simulink model "ass"  (Simulink 6.5)
settings: Solver=ode45  StartTime=0.0  StopTime=10.0  RelTol=1e-3
libraries: cdsFilt x333, cdsPhase x144, cdsRfmIO x26, cdsOsc x18, cdsMuxMatrix x8, cdsEpicsOut x3, cdsEzCaRead x1, cdsEpicsIn x1, cdsBitwise x1, cdsParameters x1
(part 12 of 17)

== system ass/PIT1/PD2_X/F3 ==
  In1 : Inport
  In2 : Inport  Port=2
  In3 : Inport  Port=3
  I : cdsFilt/Subsystem  Tag=cdsFilt  Description=|  SystemSampleTime=-1
      | Purpose:                                                                                                                                                                                                                                  
      | Standard CDS IIR filter module.                                                                                                                                                                                                           
      |                                                                                                                                                                                                                                           
      | Operation:                                                                                                                                                                                                                                
      | Consists of 10 second order section IIR filters, plus a ramped gain stage. In FE code, also provides pre-defined test points and excitation channel inputs. The filter coefficients are defined in the LIGO system using the 'foton' tool.
      |                                                                                                                                                                                                                                           
      | Usage:                                                                                                                                                                                                                                    
      | Name the part with the desired filter module name.
      settings: AttributesFormatString=%<Tag>
  PHASE : cdsPhase/Subsystem  Tag=cdsPhase  Description=Phase Rotator  SystemSampleTime=-1
      settings: AttributesFormatString=%<Tag>
  Product : Product  RndMeth=Zero
  Product1 : Product  RndMeth=Zero
  Q : cdsFilt/Subsystem  Tag=cdsFilt  Description=|  SystemSampleTime=-1
      | Purpose:                                                                                                                                                                                                                                  
      | Standard CDS IIR filter module.                                                                                                                                                                                                           
      |                                                                                                                                                                                                                                           
      | Operation:                                                                                                                                                                                                                                
      | Consists of 10 second order section IIR filters, plus a ramped gain stage. In FE code, also provides pre-defined test points and excitation channel inputs. The filter coefficients are defined in the LIGO system using the 'foton' tool.
      |                                                                                                                                                                                                                                           
      | Usage:                                                                                                                                                                                                                                    
      | Name the part with the desired filter module name.
      settings: AttributesFormatString=%<Tag>
  Terminator4 : Terminator
  Out1 : Outport
  wires:
  I/1 -> Out1/1
  PHASE/2 -> Q/1
  In1/1 -> Product/1, Product1/1
  In2/1 -> Product/2
  In3/1 -> Product1/2
  PHASE/1 -> I/1
  Product/1 -> PHASE/1
  Q/1 -> Terminator4/1
  Product1/1 -> PHASE/2

== system ass/PIT1/PD2_X/F4 ==
  In1 : Inport
  In2 : Inport  Port=2
  In3 : Inport  Port=3
  I : cdsFilt/Subsystem  Tag=cdsFilt  Description=|  SystemSampleTime=-1
      | Purpose:                                                                                                                                                                                                                                  
      | Standard CDS IIR filter module.                                                                                                                                                                                                           
      |                                                                                                                                                                                                                                           
      | Operation:                                                                                                                                                                                                                                
      | Consists of 10 second order section IIR filters, plus a ramped gain stage. In FE code, also provides pre-defined test points and excitation channel inputs. The filter coefficients are defined in the LIGO system using the 'foton' tool.
      |                                                                                                                                                                                                                                           
      | Usage:                                                                                                                                                                                                                                    
      | Name the part with the desired filter module name.
      settings: AttributesFormatString=%<Tag>
  PHASE : cdsPhase/Subsystem  Tag=cdsPhase  Description=Phase Rotator  SystemSampleTime=-1
      settings: AttributesFormatString=%<Tag>
  Product : Product  RndMeth=Zero
  Product1 : Product  RndMeth=Zero
  Q : cdsFilt/Subsystem  Tag=cdsFilt  Description=|  SystemSampleTime=-1
      | Purpose:                                                                                                                                                                                                                                  
      | Standard CDS IIR filter module.                                                                                                                                                                                                           
      |                                                                                                                                                                                                                                           
      | Operation:                                                                                                                                                                                                                                
      | Consists of 10 second order section IIR filters, plus a ramped gain stage. In FE code, also provides pre-defined test points and excitation channel inputs. The filter coefficients are defined in the LIGO system using the 'foton' tool.
      |                                                                                                                                                                                                                                           
      | Usage:                                                                                                                                                                                                                                    
      | Name the part with the desired filter module name.
      settings: AttributesFormatString=%<Tag>
  Terminator4 : Terminator
  Out1 : Outport
  wires:
  I/1 -> Out1/1
  PHASE/2 -> Q/1
  In1/1 -> Product/1, Product1/1
  In2/1 -> Product/2
  In3/1 -> Product1/2
  PHASE/1 -> I/1
  Product/1 -> PHASE/1
  Q/1 -> Terminator4/1
  Product1/1 -> PHASE/2

== system ass/PIT1/PD2_X/F5 ==
  In1 : Inport
  In2 : Inport  Port=2
  In3 : Inport  Port=3
  I : cdsFilt/Subsystem  Tag=cdsFilt  Description=|  SystemSampleTime=-1
      | Purpose:                                                                                                                                                                                                                                  
      | Standard CDS IIR filter module.                                                                                                                                                                                                           
      |                                                                                                                                                                                                                                           
      | Operation:                                                                                                                                                                                                                                
      | Consists of 10 second order section IIR filters, plus a ramped gain stage. In FE code, also provides pre-defined test points and excitation channel inputs. The filter coefficients are defined in the LIGO system using the 'foton' tool.
      |                                                                                                                                                                                                                                           
      | Usage:                                                                                                                                                                                                                                    
      | Name the part with the desired filter module name.
      settings: AttributesFormatString=%<Tag>
  PHASE : cdsPhase/Subsystem  Tag=cdsPhase  Description=Phase Rotator  SystemSampleTime=-1
      settings: AttributesFormatString=%<Tag>
  Product : Product  RndMeth=Zero
  Product1 : Product  RndMeth=Zero
  Q : cdsFilt/Subsystem  Tag=cdsFilt  Description=|  SystemSampleTime=-1
      | Purpose:                                                                                                                                                                                                                                  
      | Standard CDS IIR filter module.                                                                                                                                                                                                           
      |                                                                                                                                                                                                                                           
      | Operation:                                                                                                                                                                                                                                
      | Consists of 10 second order section IIR filters, plus a ramped gain stage. In FE code, also provides pre-defined test points and excitation channel inputs. The filter coefficients are defined in the LIGO system using the 'foton' tool.
      |                                                                                                                                                                                                                                           
      | Usage:                                                                                                                                                                                                                                    
      | Name the part with the desired filter module name.
      settings: AttributesFormatString=%<Tag>
  Terminator4 : Terminator
  Out1 : Outport
  wires:
  I/1 -> Out1/1
  PHASE/2 -> Q/1
  In1/1 -> Product/1, Product1/1
  In2/1 -> Product/2
  In3/1 -> Product1/2
  PHASE/1 -> I/1
  Product/1 -> PHASE/1
  Q/1 -> Terminator4/1
  Product1/1 -> PHASE/2

== system ass/PIT1/PD2_X/F6 ==
  In1 : Inport
  In2 : Inport  Port=2
  In3 : Inport  Port=3
  I : cdsFilt/Subsystem  Tag=cdsFilt  Description=|  SystemSampleTime=-1
      | Purpose:                                                                                                                                                                                                                                  
      | Standard CDS IIR filter module.                                                                                                                                                                                                           
      |                                                                                                                                                                                                                                           
      | Operation:                                                                                                                                                                                                                                
      | Consists of 10 second order section IIR filters, plus a ramped gain stage. In FE code, also provides pre-defined test points and excitation channel inputs. The filter coefficients are defined in the LIGO system using the 'foton' tool.
      |                                                                                                                                                                                                                                           
      | Usage:                                                                                                                                                                                                                                    
      | Name the part with the desired filter module name.
      settings: AttributesFormatString=%<Tag>
  PHASE : cdsPhase/Subsystem  Tag=cdsPhase  Description=Phase Rotator  SystemSampleTime=-1
      settings: AttributesFormatString=%<Tag>
  Product : Product  RndMeth=Zero
  Product1 : Product  RndMeth=Zero
  Q : cdsFilt/Subsystem  Tag=cdsFilt  Description=|  SystemSampleTime=-1
      | Purpose:                                                                                                                                                                                                                                  
      | Standard CDS IIR filter module.                                                                                                                                                                                                           
      |                                                                                                                                                                                                                                           
      | Operation:                                                                                                                                                                                                                                
      | Consists of 10 second order section IIR filters, plus a ramped gain stage. In FE code, also provides pre-defined test points and excitation channel inputs. The filter coefficients are defined in the LIGO system using the 'foton' tool.
      |                                                                                                                                                                                                                                           
      | Usage:                                                                                                                                                                                                                                    
      | Name the part with the desired filter module name.
      settings: AttributesFormatString=%<Tag>
  Terminator4 : Terminator
  Out1 : Outport
  wires:
  I/1 -> Out1/1
  PHASE/2 -> Q/1
  In1/1 -> Product/1, Product1/1
  In2/1 -> Product/2
  In3/1 -> Product1/2
  PHASE/1 -> I/1
  Product/1 -> PHASE/1
  Q/1 -> Terminator4/1
  Product1/1 -> PHASE/2

== system ass/PIT1/PD2_X/F7 ==
  In1 : Inport
  In2 : Inport  Port=2
  In3 : Inport  Port=3
  I : cdsFilt/Subsystem  Tag=cdsFilt  Description=|  SystemSampleTime=-1
      | Purpose:                                                                                                                                                                                                                                  
      | Standard CDS IIR filter module.                                                                                                                                                                                                           
      |                                                                                                                                                                                                                                           
      | Operation:                                                                                                                                                                                                                                
      | Consists of 10 second order section IIR filters, plus a ramped gain stage. In FE code, also provides pre-defined test points and excitation channel inputs. The filter coefficients are defined in the LIGO system using the 'foton' tool.
      |                                                                                                                                                                                                                                           
      | Usage:                                                                                                                                                                                                                                    
      | Name the part with the desired filter module name.
      settings: AttributesFormatString=%<Tag>
  PHASE : cdsPhase/Subsystem  Tag=cdsPhase  Description=Phase Rotator  SystemSampleTime=-1
      settings: AttributesFormatString=%<Tag>
  Product : Product  RndMeth=Zero
  Product1 : Product  RndMeth=Zero
  Q : cdsFilt/Subsystem  Tag=cdsFilt  Description=|  SystemSampleTime=-1
      | Purpose:                                                                                                                                                                                                                                  
      | Standard CDS IIR filter module.                                                                                                                                                                                                           
      |                                                                                                                                                                                                                                           
      | Operation:                                                                                                                                                                                                                                
      | Consists of 10 second order section IIR filters, plus a ramped gain stage. In FE code, also provides pre-defined test points and excitation channel inputs. The filter coefficients are defined in the LIGO system using the 'foton' tool.
      |                                                                                                                                                                                                                                           
      | Usage:                                                                                                                                                                                                                                    
      | Name the part with the desired filter module name.
      settings: AttributesFormatString=%<Tag>
  Terminator4 : Terminator
  Out1 : Outport
  wires:
  I/1 -> Out1/1
  PHASE/2 -> Q/1
  In1/1 -> Product/1, Product1/1
  In2/1 -> Product/2
  In3/1 -> Product1/2
  PHASE/1 -> I/1
  Product/1 -> PHASE/1
  Q/1 -> Terminator4/1
  Product1/1 -> PHASE/2

== system ass/PIT1/PD2_X/F8 ==
  In1 : Inport
  In2 : Inport  Port=2
  In3 : Inport  Port=3
  I : cdsFilt/Subsystem  Tag=cdsFilt  Description=|  SystemSampleTime=-1
      | Purpose:                                                                                                                                                                                                                                  
      | Standard CDS IIR filter module.                                                                                                                                                                                                           
      |                                                                                                                                                                                                                                           
      | Operation:                                                                                                                                                                                                                                
      | Consists of 10 second order section IIR filters, plus a ramped gain stage. In FE code, also provides pre-defined test points and excitation channel inputs. The filter coefficients are defined in the LIGO system using the 'foton' tool.
      |                                                                                                                                                                                                                                           
      | Usage:                                                                                                                                                                                                                                    
      | Name the part with the desired filter module name.
      settings: AttributesFormatString=%<Tag>
  PHASE : cdsPhase/Subsystem  Tag=cdsPhase  Description=Phase Rotator  SystemSampleTime=-1
      settings: AttributesFormatString=%<Tag>
  Product : Product  RndMeth=Zero
  Product1 : Product  RndMeth=Zero
  Q : cdsFilt/Subsystem  Tag=cdsFilt  Description=|  SystemSampleTime=-1
      | Purpose:                                                                                                                                                                                                                                  
      | Standard CDS IIR filter module.                                                                                                                                                                                                           
      |                                                                                                                                                                                                                                           
      | Operation:                                                                                                                                                                                                                                
      | Consists of 10 second order section IIR filters, plus a ramped gain stage. In FE code, also provides pre-defined test points and excitation channel inputs. The filter coefficients are defined in the LIGO system using the 'foton' tool.
      |                                                                                                                                                                                                                                           
      | Usage:                                                                                                                                                                                                                                    
      | Name the part with the desired filter module name.
      settings: AttributesFormatString=%<Tag>
  Terminator4 : Terminator
  Out1 : Outport
  wires:
  I/1 -> Out1/1
  PHASE/2 -> Q/1
  In1/1 -> Product/1, Product1/1
  In2/1 -> Product/2
  In3/1 -> Product1/2
  PHASE/1 -> I/1
  Product/1 -> PHASE/1
  Q/1 -> Terminator4/1
  Product1/1 -> PHASE/2

== system ass/PIT1/PD2_X/F9 ==
  In1 : Inport
  In2 : Inport  Port=2
  In3 : Inport  Port=3
  I : cdsFilt/Subsystem  Tag=cdsFilt  Description=|  SystemSampleTime=-1
      | Purpose:                                                                                                                                                                                                                                  
      | Standard CDS IIR filter module.                                                                                                                                                                                                           
      |                                                                                                                                                                                                                                           
      | Operation:                                                                                                                                                                                                                                
      | Consists of 10 second order section IIR filters, plus a ramped gain stage. In FE code, also provides pre-defined test points and excitation channel inputs. The filter coefficients are defined in the LIGO system using the 'foton' tool.
      |                                                                                                                                                                                                                                           
      | Usage:                                                                                                                                                                                                                                    
      | Name the part with the desired filter module name.
      settings: AttributesFormatString=%<Tag>
  PHASE : cdsPhase/Subsystem  Tag=cdsPhase  Description=Phase Rotator  SystemSampleTime=-1
      settings: AttributesFormatString=%<Tag>
  Product : Product  RndMeth=Zero
  Product1 : Product  RndMeth=Zero
  Q : cdsFilt/Subsystem  Tag=cdsFilt  Description=|  SystemSampleTime=-1
      | Purpose:                                                                                                                                                                                                                                  
      | Standard CDS IIR filter module.                                                                                                                                                                                                           
      |                                                                                                                                                                                                                                           
      | Operation:                                                                                                                                                                                                                                
      | Consists of 10 second order section IIR filters, plus a ramped gain stage. In FE code, also provides pre-defined test points and excitation channel inputs. The filter coefficients are defined in the LIGO system using the 'foton' tool.
      |                                                                                                                                                                                                                                           
      | Usage:                                                                                                                                                                                                                                    
      | Name the part with the desired filter module name.
      settings: AttributesFormatString=%<Tag>
  Terminator4 : Terminator
  Out1 : Outport
  wires:
  I/1 -> Out1/1
  PHASE/2 -> Q/1
  In1/1 -> Product/1, Product1/1
  In2/1 -> Product/2
  In3/1 -> Product1/2
  PHASE/1 -> I/1
  Product/1 -> PHASE/1
  Q/1 -> Terminator4/1
  Product1/1 -> PHASE/2

== system ass/PIT1/PD3_X/F1 ==
  In1 : Inport
  In2 : Inport  Port=2
  In3 : Inport  Port=3
  I : cdsFilt/Subsystem  Tag=cdsFilt  Description=|  SystemSampleTime=-1
      | Purpose:                                                                                                                                                                                                                                  
      | Standard CDS IIR filter module.                                                                                                                                                                                                           
      |                                                                                                                                                                                                                                           
      | Operation:                                                                                                                                                                                                                                
      | Consists of 10 second order section IIR filters, plus a ramped gain stage. In FE code, also provides pre-defined test points and excitation channel inputs. The filter coefficients are defined in the LIGO system using the 'foton' tool.
      |                                                                                                                                                                                                                                           
      | Usage:                                                                                                                                                                                                                                    
      | Name the part with the desired filter module name.
      settings: AttributesFormatString=%<Tag>
  PHASE : cdsPhase/Subsystem  Tag=cdsPhase  Description=Phase Rotator  SystemSampleTime=-1
      settings: AttributesFormatString=%<Tag>
  Product : Product  RndMeth=Zero
  Product1 : Product  RndMeth=Zero
  Q : cdsFilt/Subsystem  Tag=cdsFilt  Description=|  SystemSampleTime=-1
      | Purpose:                                                                                                                                                                                                                                  
      | Standard CDS IIR filter module.                                                                                                                                                                                                           
      |                                                                                                                                                                                                                                           
      | Operation:                                                                                                                                                                                                                                
      | Consists of 10 second order section IIR filters, plus a ramped gain stage. In FE code, also provides pre-defined test points and excitation channel inputs. The filter coefficients are defined in the LIGO system using the 'foton' tool.
      |                                                                                                                                                                                                                                           
      | Usage:                                                                                                                                                                                                                                    
      | Name the part with the desired filter module name.
      settings: AttributesFormatString=%<Tag>
  Terminator4 : Terminator
  Out1 : Outport
  wires:
  I/1 -> Out1/1
  PHASE/2 -> Q/1
  In1/1 -> Product/1, Product1/1
  In2/1 -> Product/2
  In3/1 -> Product1/2
  PHASE/1 -> I/1
  Product/1 -> PHASE/1
  Q/1 -> Terminator4/1
  Product1/1 -> PHASE/2

== system ass/PIT1/PD3_X/F2 ==
  In1 : Inport
  In2 : Inport  Port=2
  In3 : Inport  Port=3
  I : cdsFilt/Subsystem  Tag=cdsFilt  Description=|  SystemSampleTime=-1
      | Purpose:                                                                                                                                                                                                                                  
      | Standard CDS IIR filter module.                                                                                                                                                                                                           
      |                                                                                                                                                                                                                                           
      | Operation:                                                                                                                                                                                                                                
      | Consists of 10 second order section IIR filters, plus a ramped gain stage. In FE code, also provides pre-defined test points and excitation channel inputs. The filter coefficients are defined in the LIGO system using the 'foton' tool.
      |                                                                                                                                                                                                                                           
      | Usage:                                                                                                                                                                                                                                    
      | Name the part with the desired filter module name.
      settings: AttributesFormatString=%<Tag>
  PHASE : cdsPhase/Subsystem  Tag=cdsPhase  Description=Phase Rotator  SystemSampleTime=-1
      settings: AttributesFormatString=%<Tag>
  Product : Product  RndMeth=Zero
  Product1 : Product  RndMeth=Zero
  Q : cdsFilt/Subsystem  Tag=cdsFilt  Description=|  SystemSampleTime=-1
      | Purpose:                                                                                                                                                                                                                                  
      | Standard CDS IIR filter module.                                                                                                                                                                                                           
      |                                                                                                                                                                                                                                           
      | Operation:                                                                                                                                                                                                                                
      | Consists of 10 second order section IIR filters, plus a ramped gain stage. In FE code, also provides pre-defined test points and excitation channel inputs. The filter coefficients are defined in the LIGO system using the 'foton' tool.
      |                                                                                                                                                                                                                                           
      | Usage:                                                                                                                                                                                                                                    
      | Name the part with the desired filter module name.
      settings: AttributesFormatString=%<Tag>
  Terminator4 : Terminator
  Out1 : Outport
  wires:
  I/1 -> Out1/1
  PHASE/2 -> Q/1
  In1/1 -> Product/1, Product1/1
  In2/1 -> Product/2
  In3/1 -> Product1/2
  PHASE/1 -> I/1
  Product/1 -> PHASE/1
  Q/1 -> Terminator4/1
  Product1/1 -> PHASE/2

== system ass/PIT1/PD3_X/F3 ==
  In1 : Inport
  In2 : Inport  Port=2
  In3 : Inport  Port=3
  I : cdsFilt/Subsystem  Tag=cdsFilt  Description=|  SystemSampleTime=-1
      | Purpose:                                                                                                                                                                                                                                  
      | Standard CDS IIR filter module.                                                                                                                                                                                                           
      |                                                                                                                                                                                                                                           
      | Operation:                                                                                                                                                                                                                                
      | Consists of 10 second order section IIR filters, plus a ramped gain stage. In FE code, also provides pre-defined test points and excitation channel inputs. The filter coefficients are defined in the LIGO system using the 'foton' tool.
      |                                                                                                                                                                                                                                           
      | Usage:                                                                                                                                                                                                                                    
      | Name the part with the desired filter module name.
      settings: AttributesFormatString=%<Tag>
  PHASE : cdsPhase/Subsystem  Tag=cdsPhase  Description=Phase Rotator  SystemSampleTime=-1
      settings: AttributesFormatString=%<Tag>
  Product : Product  RndMeth=Zero
  Product1 : Product  RndMeth=Zero
  Q : cdsFilt/Subsystem  Tag=cdsFilt  Description=|  SystemSampleTime=-1
      | Purpose:                                                                                                                                                                                                                                  
      | Standard CDS IIR filter module.                                                                                                                                                                                                           
      |                                                                                                                                                                                                                                           
      | Operation:                                                                                                                                                                                                                                
      | Consists of 10 second order section IIR filters, plus a ramped gain stage. In FE code, also provides pre-defined test points and excitation channel inputs. The filter coefficients are defined in the LIGO system using the 'foton' tool.
      |                                                                                                                                                                                                                                           
      | Usage:                                                                                                                                                                                                                                    
      | Name the part with the desired filter module name.
      settings: AttributesFormatString=%<Tag>
  Terminator4 : Terminator
  Out1 : Outport
  wires:
  I/1 -> Out1/1
  PHASE/2 -> Q/1
  In1/1 -> Product/1, Product1/1
  In2/1 -> Product/2
  In3/1 -> Product1/2
  PHASE/1 -> I/1
  Product/1 -> PHASE/1
  Q/1 -> Terminator4/1
  Product1/1 -> PHASE/2

== system ass/PIT1/PD3_X/F4 ==
  In1 : Inport
  In2 : Inport  Port=2
  In3 : Inport  Port=3
  I : cdsFilt/Subsystem  Tag=cdsFilt  Description=|  SystemSampleTime=-1
      | Purpose:                                                                                                                                                                                                                                  
      | Standard CDS IIR filter module.                                                                                                                                                                                                           
      |                                                                                                                                                                                                                                           
      | Operation:                                                                                                                                                                                                                                
      | Consists of 10 second order section IIR filters, plus a ramped gain stage. In FE code, also provides pre-defined test points and excitation channel inputs. The filter coefficients are defined in the LIGO system using the 'foton' tool.
      |                                                                                                                                                                                                                                           
      | Usage:                                                                                                                                                                                                                                    
      | Name the part with the desired filter module name.
      settings: AttributesFormatString=%<Tag>
  PHASE : cdsPhase/Subsystem  Tag=cdsPhase  Description=Phase Rotator  SystemSampleTime=-1
      settings: AttributesFormatString=%<Tag>
  Product : Product  RndMeth=Zero
  Product1 : Product  RndMeth=Zero
  Q : cdsFilt/Subsystem  Tag=cdsFilt  Description=|  SystemSampleTime=-1
      | Purpose:                                                                                                                                                                                                                                  
      | Standard CDS IIR filter module.                                                                                                                                                                                                           
      |                                                                                                                                                                                                                                           
      | Operation:                                                                                                                                                                                                                                
      | Consists of 10 second order section IIR filters, plus a ramped gain stage. In FE code, also provides pre-defined test points and excitation channel inputs. The filter coefficients are defined in the LIGO system using the 'foton' tool.
      |                                                                                                                                                                                                                                           
      | Usage:                                                                                                                                                                                                                                    
      | Name the part with the desired filter module name.
      settings: AttributesFormatString=%<Tag>
  Terminator4 : Terminator
  Out1 : Outport
  wires:
  I/1 -> Out1/1
  PHASE/2 -> Q/1
  In1/1 -> Product/1, Product1/1
  In2/1 -> Product/2
  In3/1 -> Product1/2
  PHASE/1 -> I/1
  Product/1 -> PHASE/1
  Q/1 -> Terminator4/1
  Product1/1 -> PHASE/2
